simulink model "sim_ieee"  (R2014b)
settings: Solver=ode113  StartTime=0.0  StopTime=20  RelTol=1e-3
values from neighbouring files (symbols this model uses):
  k1 = .00001    (= 1e-05)    [faragasso_params.m]
  k2 = .00023    (= 0.00023)    [faragasso_params.m]
  k3 = .000187    (= 0.000187)    [faragasso_params.m]
  kp = 1.1    [faragasso_params.m]
  theta0 = 0    [faragasso_params.m]
  v = 5    [faragasso_params.m]
  x0 = .25    (= 0.25)    [faragasso_params.m]
  y0 = 0    [faragasso_params.m]
undefined symbols (not defined in the file or in its folder): mfun, sigbuilder_block
settings Model: Creator=root  LastModifiedBy=root
settings SolverCC: AutoInsertRateTranBlk=on

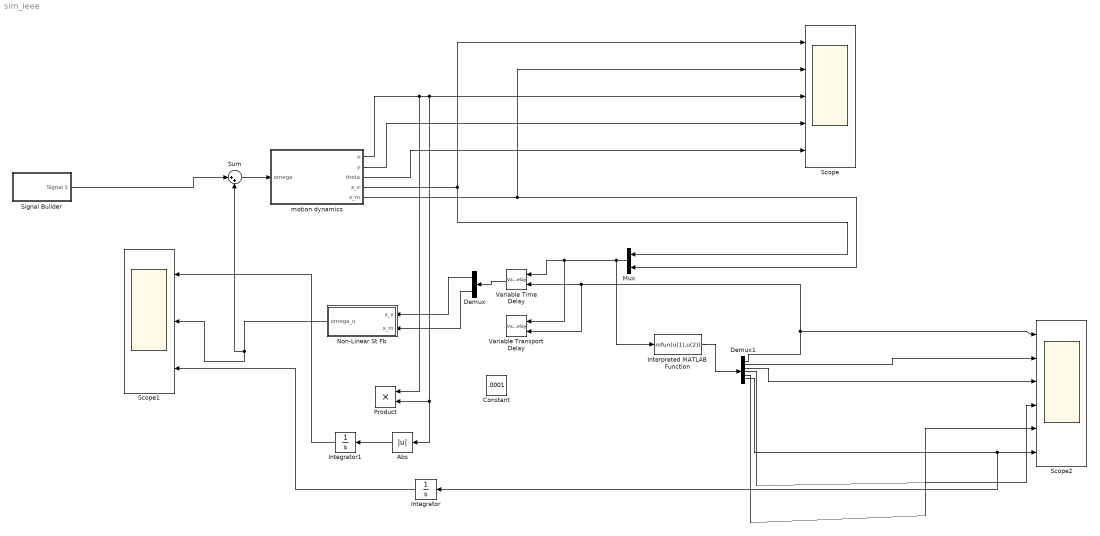
== system sim_ieee ==
  Abs : Abs
  Constant : Constant  Value=.0001
  Demux : Demux  Outputs=2
  Demux1 : Demux  Outputs=6
  Integrator : Integrator
  Integrator1 : Integrator
  Interpreted MATLAB Function : MATLABFcn  MATLABFcn=mfun(u(1),u(2))  OutputSignalType=real  Output1D=off
  Mux : Mux  Inputs=2
  Non-Linear St Fb : Subsystem
  Product : Product
  Scope : Scope  NumInputPorts=5
      settings: TimeRange=20  YMin=-2e-07~-9.999999999999999e-06~-0.05~0~-0.02  YMax=1e-07~3e-05~0.1~100~0.009999999999999998  SaveName=SysOut
  Scope1 : Scope  NumInputPorts=3
      settings: YMin=-5~-5~-5  YMax=5~5~5  SampleTime=0.001
  Scope2 : Scope  NumInputPorts=6
      settings: TimeRange=20  YMin=-1~5~5~-1~-1~5  YMax=2~7~7~1~1~8  SaveName=Scheduler  SampleInput=on
  Signal Builder : Subsystem  Tag=STV Subsys  LoadFcn=sigbuilder_block('load');  StartFcn=sigbuilder_block('start');  StopFcn=sigbuilder_block('stop');  ClipboardFcn=sigbuilder_block('clipboard');  mask(Sigbuilder block){}
      mask help: Simulink:masks:SigbuilderBlock_MD
      mask init:
      | if ~strcmp(get_param(bdroot(gcbh),'SimulationStatus'),'stopped') tuvar = sigbuilder_block('maskInit'); end
      settings: CopyFcn=sigbuilder_block('copy');  DeleteFcn=sigbuilder_block('delete');  ModelCloseFcn=sigbuilder_block('modelClose');  PreSaveFcn=sigbuilder_block('preSave');  PauseFcn=sigbuilder_block('pause');  ContinueFcn=sigbuilder_block('continue');  NameChangeFcn=sigbuilder_block('namechange');  OpenFcn=sigbuilder_block('open',[437.6 199.2 550.4 400 ]);  CloseFcn=sigbuilder_block('close');
      mask Display: plot(0, 0, 100, 100,[2, 2, 32, 32, 2], [68, 8, 8, 68, 68],[32, 2], [38, 38], [32, 19, 2],[53, 60, 44], [32, 17, 17, 2],[16, 16, 31, 31]);txt = getActiveGroup(gcbh);text(2, 100, txt,'verticalAlignment', 'top');
  Sum : Sum  Inputs=|++
  Variable Time Delay : VariableTransportDelay  MaximumDelay=10  FixedBuffer=on  ZeroDelay=on  TransDelayFeedthrough=on  PadeOrder=2
  Variable Transport Delay : VariableTransportDelay  VariableDelayType=Variable transport delay  MaximumDelay=10
  motion dynamics : Subsystem
  wires:
  motion dynamics/1(x) -> Product/1, Abs/1, Product/2, Scope/3
  motion dynamics/3(theta) -> Scope/5
  motion dynamics/2(y) -> Scope/4
  motion dynamics/5(x_m) -> Mux/2, Scope/2
  Non-Linear St Fb/1(omega_u) -> Sum/2, Scope1/2
  motion dynamics/4(x_v) -> Scope/1, Mux/1
  Sum/1 -> motion dynamics/1(omega)
  Mux/1 -> Interpreted MATLAB Function/1, Variable Transport Delay/1, Variable Time Delay/1
  Demux/1 -> Non-Linear St Fb/1(x_v)
  Demux/2 -> Non-Linear St Fb/2(x_m)
  Signal Builder/1(Signal 1) -> Sum/1
  Interpreted MATLAB Function/1 -> Demux1/1
  Demux1/1 -> Variable Transport Delay/2, Variable Time Delay/2, Scope2/1
  Demux1/2 -> Scope2/2
  Demux1/3 -> Scope2/3
  Demux1/4 -> Scope2/4
  Demux1/5 -> Scope2/5
  Demux1/6 -> Integrator/1, Scope2/6
  Integrator/1 -> Scope1/3
  Integrator1/1 -> Scope1/1
  Abs/1 -> Integrator1/1
  Variable Time Delay/1 -> Demux/1

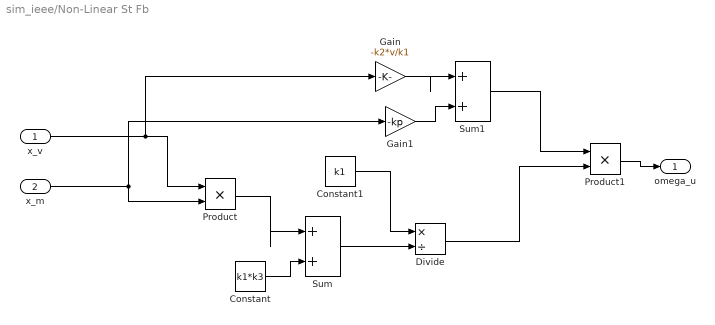
== system sim_ieee/Non-Linear St Fb ==
  x_v : Inport
  x_m : Inport  Port=2
  Constant : Constant  Value=k1*k3
  Constant1 : Constant  Value=k1
  Divide : Product  Inputs=*/
  Gain : Gain  Gain=-k2*v/k1
  Gain1 : Gain  Gain=-kp
  Product : Product
  Product1 : Product
  Sum : Sum  Inputs=|++
  Sum1 : Sum  Inputs=|++
  omega_u : Outport
  wires:
  Constant/1 -> Sum/2
  Sum/1 -> Divide/2
  x_v/1 -> Gain/1, Product/1
  x_m/1 -> Product/2, Gain1/1
  Product/1 -> Sum/1
  Constant1/1 -> Divide/1
  Gain/1 -> Sum1/1
  Gain1/1 -> Sum1/2
  Sum1/1 -> Product1/1
  Divide/1 -> Product1/2
  Product1/1 -> omega_u/1

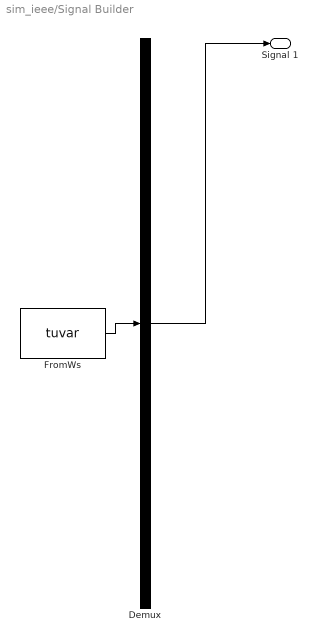
== system sim_ieee/Signal Builder ==
  Demux : Demux  Tag=STV Demux  Outputs=1
  FromWs : FromWorkspace  Tag=STV FromWs  VariableName=tuvar  SampleTime=0
      SigBuilderData=|
      | common.afterFinalStr = 'Extrapolate'
      | common.sampleTime = 0
      | dataSet.timeRange = [0 20]
      | dataSet.name = 'Group 1'
      | sbobj.Groups.Name = 'Group 1'
      | sbobj.Groups.Signals.Name = 'Signal 1'
      | sbobj.Groups.Signals.XData = [0 10 10 12 12 20]
      | sbobj.Groups.Signals.YData = [0 0 0.05 0.05 0 0]
      | sbobj.Groups.TimeRange = [0 20]
  Signal 1 : Outport  Tag=STV Outport
  wires:
  Demux/1 -> Signal 1/1
  FromWs/1 -> Demux/1

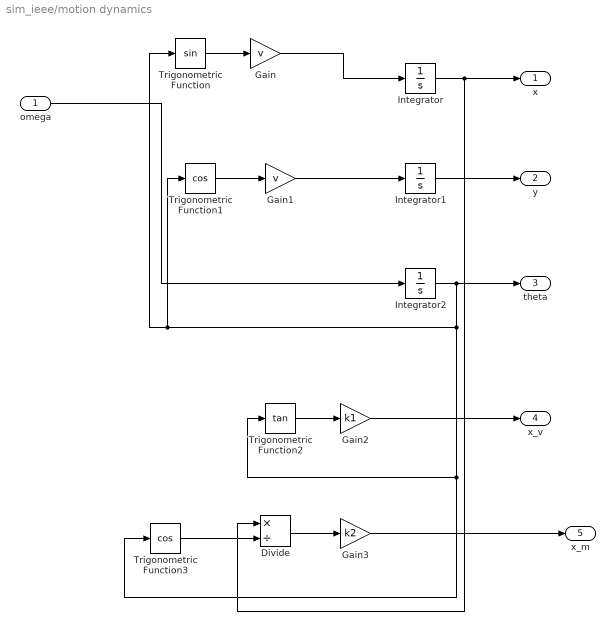
== system sim_ieee/motion dynamics ==
  omega : Inport
  Divide : Product  Inputs=*/
  Gain : Gain  Gain=v
  Gain1 : Gain  Gain=v
  Gain2 : Gain  Gain=k1
  Gain3 : Gain  Gain=k2
  Integrator : Integrator  InitialCondition=x0
  Integrator1 : Integrator  InitialCondition=y0
  Integrator2 : Integrator  InitialCondition=theta0
  Trigonometric Function : Trigonometry
  Trigonometric Function1 : Trigonometry  Operator=cos
  Trigonometric Function2 : Trigonometry  Operator=tan
  Trigonometric Function3 : Trigonometry  Operator=cos
  x : Outport
  y : Outport  Port=2
  theta : Outport  Port=3
  x_v : Outport  Port=4
  x_m : Outport  Port=5
  wires:
  Integrator2/1 -> Trigonometric Function3/1, Trigonometric Function2/1, Trigonometric Function/1, Trigonometric Function1/1, theta/1
  Trigonometric Function/1 -> Gain/1
  Gain/1 -> Integrator/1
  Integrator/1 -> Divide/1, x/1
  Trigonometric Function1/1 -> Gain1/1
  Gain1/1 -> Integrator1/1
  Integrator1/1 -> y/1
  omega/1 -> Integrator2/1
  Trigonometric Function2/1 -> Gain2/1
  Gain2/1 -> x_v/1
  Trigonometric Function3/1 -> Divide/2
  Divide/1 -> Gain3/1
  Gain3/1 -> x_m/1
